simulink model "untitled"  (Simulink 5.0)
settings: Solver=ode3  StartTime=0.0  StopTime=TMAX  FixedStep=Ta  RelTol=1e-3
values from neighbouring files (symbols this model uses):
  A = 30    [aula1304.m]    (also in script_controle_lr.m = [1/p 1; (1+z/p) z])
  den = Gs.Den{1}    [aula1304.m]
  Kd = 0    [aula1304.m]
  Ki = 0    [aula1304.m]
  Kp = 12    [aula1304.m]
  LOWER_SAT = -5    [aula1304.m]
  MEDIA_RUIDO = 0    [aula1304.m]
  num = Gs.Num{1}    [aula1304.m]
  Tau_d = 1/200    (= 0.005)    [aula1304.m]
  UPPER_SAT = 5    [aula1304.m]
  VARIANCIA_RUIDO = 0.05    [aula1304.m]
settings Model: LastModifiedBy=ENGENHARIA

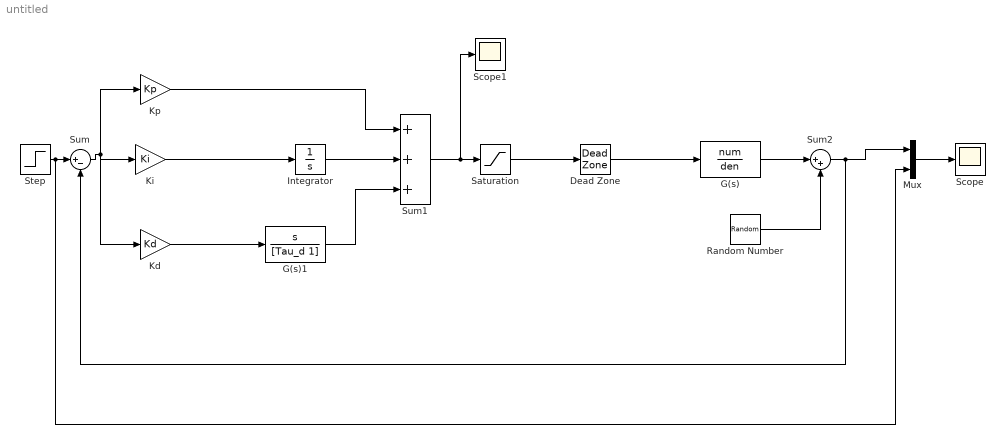
== system untitled ==
  Dead Zone : DeadZone  LowerValue=START_DEAD_ZONE  UpperValue=END_DEAD_ZONE  SaturateOnIntegerOverflow=on
  G(s) : TransferFcn  Numerator=num  Denominator=den
  G(s)1 : TransferFcn  Numerator=[1 0]  Denominator=[Tau_d 1]
  Integrator : Integrator
  Kd : Gain  Gain=Kd  SaturateOnIntegerOverflow=on
  Ki : Gain  Gain=Ki  SaturateOnIntegerOverflow=on
  Kp : Gain  Gain=Kp  SaturateOnIntegerOverflow=on
  Mux : Mux  Inputs=2
  Random Number : RandomNumber  Mean=MEDIA_RUIDO  Variance=VARIANCIA_RUIDO  SampleTime=0
  Saturation : Saturate  UpperLimit=UPPER_SAT  LowerLimit=LOWER_SAT
  Scope : Scope
      settings: SaveName=sinais  DataFormat=Array
  Scope1 : Scope
      settings: TimeRange=10  YMin=-1
  Step : Step  Time=0  After=A  SampleTime=0
  Sum : Sum  Inputs=|+-  SaturateOnIntegerOverflow=on
  Sum1 : Sum  Inputs=+++  SaturateOnIntegerOverflow=on
  Sum2 : Sum  Inputs=|++  SaturateOnIntegerOverflow=on
  wires:
  Saturation/1 -> Dead Zone/1
  Dead Zone/1 -> G(s)/1
  Step/1 -> Sum/1, Mux/2
  Kp/1 -> Sum1/1
  Integrator/1 -> Sum1/2
  Ki/1 -> Integrator/1
  Kd/1 -> G(s)1/1
  Sum/1 -> Kp/1, Kd/1, Ki/1
  Sum1/1 -> Saturation/1, Scope1/1
  Mux/1 -> Scope/1
  G(s)/1 -> Sum2/1
  Random Number/1 -> Sum2/2
  Sum2/1 -> Mux/1, Sum/2
  G(s)1/1 -> Sum1/3
